simulink model "statemodel"  (R2018b)
settings: Solver=ode45  StartTime=0.0  StopTime=10.0  RelTol=1e-3  AbsTol=1e-6
values from neighbouring files (symbols this model uses):
  C = [1 0; 0 1; 1 -R; 0 R; 0 -1]    [circex.m]
  L = y * 100e-3    (= 1)    [circex.m]
  R = z    (= 10)    [circex.m]
settings Model: ExtModeTrigMode=oneshot  ExtModeArmWhenConnect=off  Creator=eechris  LastModifiedBy=eechris
settings DataIOCC: SaveFormat=Array  SignalLoggingSaveFormat=ModelDataLogs
settings OptimizationCC: BlockReduction=off  BooleanDataType=off
settings DebuggingCC: SaveWithParameterizedLinksMsg=none  UnderspecifiedInitializationDetection=Classic  MergeDetectMultiDrivingBlocksExec=none  SignalResolutionControl=TryResolveAllWithWarning  MultiTaskDSMMsg=warning  MultiTaskCondExecSysMsg=none
settings HardwareCC: TargetUnknown=on
settings ModelReferenceCC: PropagateSignalLabelsOutOfModel=off
settings GRTTargetCC: CombineOutputUpdateFcns=off  GRTInterface=on

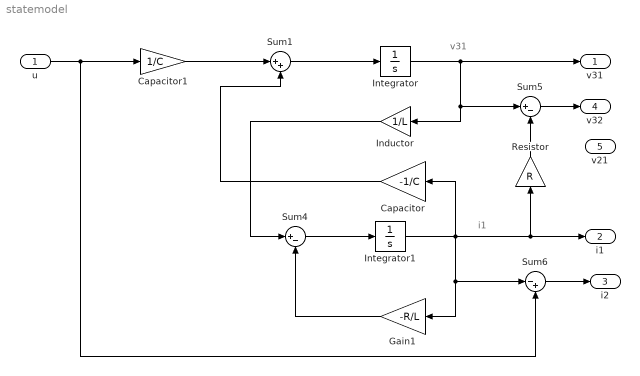
== system statemodel ==
  note: v31
  note: i1
  u : Inport
  Capacitor : Gain  Gain=-1/C  SaturateOnIntegerOverflow=on  OutDataTypeStr=Inherit: Same as input  ParamDataTypeStr=Inherit: Same as input
  Capacitor1 : Gain  Gain=1/C  SaturateOnIntegerOverflow=on  OutDataTypeStr=Inherit: Same as input  ParamDataTypeStr=Inherit: Same as input
  Gain1 : Gain  Gain=-R/L  SaturateOnIntegerOverflow=on  OutDataTypeStr=Inherit: Same as input  ParamDataTypeStr=Inherit: Same as input
  Inductor : Gain  Gain=1/L  SaturateOnIntegerOverflow=on  OutDataTypeStr=Inherit: Same as input  ParamDataTypeStr=Inherit: Same as input
  Integrator : Integrator
  Integrator1 : Integrator
  Resistor : Gain  Gain=R  SaturateOnIntegerOverflow=on  OutDataTypeStr=Inherit: Same as input  ParamDataTypeStr=Inherit: Same as input
  Sum1 : Sum  Inputs=|++  SaturateOnIntegerOverflow=on  InputSameDT=on  OutDataTypeStr=Inherit: Same as first input
  Sum4 : Sum  Inputs=|+-  SaturateOnIntegerOverflow=on  InputSameDT=on  OutDataTypeStr=Inherit: Same as first input
  Sum5 : Sum  Inputs=|+-  SaturateOnIntegerOverflow=on  InputSameDT=on  OutDataTypeStr=Inherit: Same as first input
  Sum6 : Sum  Inputs=|-+  SaturateOnIntegerOverflow=on  InputSameDT=on  OutDataTypeStr=Inherit: Same as first input
  v31 : Outport
  i1 : Outport  Port=2
  i2 : Outport  Port=3
  v32 : Outport  Port=4
  v21 : Outport  Port=5
  wires:
  Sum4/1 -> Integrator1/1
  Integrator1/1 -> Capacitor/1, i1/1, Resistor/1, Gain1/1, Sum6/1
  Capacitor/1 -> Sum1/2
  Sum1/1 -> Integrator/1
  Integrator/1 -> v31/1, Inductor/1, Sum5/1
  Sum6/1 -> i2/1
  Sum5/1 -> v32/1
  Capacitor1/1 -> Sum1/1
  Gain1/1 -> Sum4/2
  Inductor/1 -> Sum4/1
  Resistor/1 -> Sum5/2
  u/1 -> Capacitor1/1, Sum6/2
